simulink model "sim_all"  (R2020a)
settings: Solver=VariableStepAuto  StartTime=0.0  StopTime=2000  RelTol=1e-3
undefined symbols (not defined in the file or in its folder): a1, a2, alpha1, alpha2, cornerA, cornerB, cornerC, cornerD, ctrl_clockwise, ctrl_int_bound_or, ctrl_int_bound_pos, ctrl_k_or, ctrl_k_pos, ctrl_Ki_vel, ctrl_Kp_v_pos, ctrl_Kp_vel, ctrl_TAM, ctrl_Ts, ctrl_va_uncontrolled, ctrl_vel_uncontrolled, D, dead_zone_limit, depth, DiscIntNeverNeededParam, distanceFromWall, initInspectedSide, initPoint, mod_A, mod_Cd_F, mod_Cd_M, mod_eta_init, mod_g, mod_h0, mod_Ixx, mod_Iyy, mod_Izz, mod_Kp_dot, mod_lat0, mod_lon0, mod_m, mod_Mq_dot, mod_ni_init, mod_Nr_dot, mod_p1, mod_p2, mod_p3, mod_p4, mod_p5, mod_p6, mod_R, mod_Rm, mod_t1, mod_t2, mod_t3, mod_t4, mod_t5, mod_t6, mod_W, mod_Xu_dot, mod_Yv_dot ... (+53)
libraries: simulink x8, cstblocks x6, simulink_extras x1
(part 5 of 6)

== matlab function sim_all/Controller_mk4_v3/Mixer/Mix ==
  data: Tp input; T output; Tv input; To input; ctrl_T_max parameter
%% funzione che permette di gestire le saturazioni dei motori
function T = Mix(Tp, Tv, To, ctrl_T_max)
    T_sat = [   ctrl_T_max   ctrl_T_max   ctrl_T_max   ctrl_T_max   ctrl_T_max   ctrl_T_max;...
               -ctrl_T_max  -ctrl_T_max  -ctrl_T_max  -ctrl_T_max  -ctrl_T_max  -ctrl_T_max];
    tmp = Tp + Tv + To;
    freg = sumSat(ctrl_T_max, tmp);                 % freg indica se il vettore è da regolare
    if freg == true
        if sumSat(ctrl_T_max, To+Tp) == false       % caso in cui To+Tp non satura
            T_tmp = To + Tp;
            [T_sat, T_new] = prior(T_sat, T_tmp);
            [T_sat, T_new] = prior(T_sat, Tv);
            T = T_tmp + T_new;
        else                                        % caso generale, ridimensiona tutti i vettori che fanno saturare
            T_tmp = 0;
            [T_sat, T_new] = prior(T_sat, To);
            T_tmp = T_tmp + T_new;
            [T_sat, T_new] = prior(T_sat, Tp);
            T_tmp = T_tmp + T_new;
            [T_sat, T_new] = prior(T_sat, Tv);
            T = T_tmp + T_new;
        end
    else
        T = tmp;
    end
end

% sumSat() restituisce 1 se il vettore T_in supera la saturazione, è solo
% un controllo iniziale in quanto controlla solo se la somma delle spinte
% rientra in T_max
function resp = sumSat(T_max, T_in)
    tmp = false;
    for i=1:length(T_in)
        if abs(T_in(i)) > T_max
            tmp = true;
        end
    end
    resp = tmp;
end

% prior() prende vettore in ingresso e vettore delle saturazioni e
% restituisce vettore in ingresso ridimensionato e nuovo vettore delle
% saturazioni
function [T_sat_new, T_reg] = prior(T_sat, T_new)
    T_sat_tmp = T_sat;
    recalc = false;                 % serve per sapere se bisogna ricalcolare le precedenti saturazioni
    for i = 1:length(T_new)         % ciclo per calcolare i nuovi vettori ridimensionati
        if T_new(i)>0               % azione del motore positiva
            tmp = T_sat_tmp(1,i) - T_new(i);        % nuova saturazione temporanea
            if tmp < 0
                if i < 5                            % devo scalare i primi 4 motori per mantenere la direzione
                    k = abs(T_sat_tmp(1,i)/T_new(i));
                    T_new(1:4) = T_new(1:4) * k;
                    if i~=1                 % devo riaggiustare le T_sat precedenti se il motore che satura non è il primo
                        recalc = true;      % riaggiusto i T_sat in prior2
                    end
                else
                    k = abs(T_sat_tmp(1,i)/T_new(i));
                    j = ((floor(i/2.1)+1)*2);           % escamotage per prendere le coppie giuste, era per le coppie
                    T_new(j-1:j) = T_new(j-1:j) * k;    % ridimensiono le componenti relative al grado di libertà
                    if mod(i, 2) == 0                   % devo riaggiustare la T_sat precedente se i pari
                        recalc = true;                  % riaggiusto gli T_sat
                    end
                end
            end
            T_sat_tmp(1,i) = T_sat_tmp(1,i) - T_new(i);
            T_sat_tmp(2,i) = T_sat_tmp(2,i) - T_new(i);
        elseif T_new(i)<0                           % è identico al codice per T>0 ma speculare
            tmp = T_sat_tmp(2,i) - T_new(i);
            if tmp > 0
                if i < 5                            % devo scalare i primi 4 motori
                    k = abs(T_sat_tmp(2,i)/T_new(i));
                    T_new(1:4) = T_new(1:4) * k;
                    if i~=1                         % devo riaggiustare le T_sat precedenti se i 
                        recalc = true;              % riaggiusto gli T_sat
                    end
                else
                    k = abs(T_sat_tmp(2,i)/T_new(i));
                    j = (floor(i/2.1)+1)*2;     % escamotage per prendere le coppie giuste
                    T_new(j-1:j) = T_new(j-1:j) * k;
                    if mod(i, 2) == 0           % devo riaggiustare la T_sat precedente se i pari
                        recalc = true;          % riaggiusto gli T_sat
                    end
                end
            end
            T_sat_tmp(2,i) = T_sat_tmp(2,i) - T_new(i);
            T_sat_tmp(1,i) = T_sat_tmp(1,i) - T_new(i);
        end
    end
    if recalc == true
        % devo rifare il ciclo con i nuovi T_new
        [T_sat_tmp, T_new] = prior2(T_sat, T_new);
    end
    T_sat_new = T_sat_tmp;      % T_sat_new è il nuovo vettore delle saturazioni
    T_reg = T_new;              % T_reg è il nuovo vettore scalato
end

% prior2() aggiusta il vettore delle saturazioni T_sat, uso interno a
% prior()
function [T_sat_new, T_reg] = prior2(T_sat, T_new)
    T_sat_tmp = T_sat;
    for i = 1:length(T_new)        % ciclo per calcolare quanti giri rimanenti prima di saturare
        if T_new(i)>0              % azione del motore positiva
            tmp = T_sat_tmp(1,i) - T_new(i);       % nuova saturazione temporanea
            T_sat_tmp(1,i) = tmp;
            T_sat_tmp(2,i) = T_sat_tmp(2,i) - T_new(i);
        else
            tmp = T_sat_tmp(2,i) - T_new(i);
            T_sat_tmp(2,i) = tmp;
            T_sat_tmp(1,i) = T_sat_tmp(1,i) - T_new(i);
        end
    end
    T_sat_new = T_sat_tmp;
    T_reg = T_new;
end

== matlab function sim_all/Mission_supervisor_v3/Mission_Supervisor/MATLAB Function1 ==
  data: punto_iniz_patt output size=3; initInspectedSide parameter; distanceFromWall parameter; initPoint parameter; Or_in output; dps_fin output; cornerA parameter; cornerB parameter; cornerC parameter; cornerD parameter; relativeDirection parameter; alfa output
function [punto_iniz_patt, Or_in, dps_fin, alfa] = ambiente(initInspectedSide,distanceFromWall,initPoint,cornerA, cornerB, cornerC, cornerD, relativeDirection)
 
    %% Unità di misura 
    
    % punto_iniz_patt, initPoint, cornerA, cornerB, cornerC, cornerD        [deg, deg, m]
    % Or_in                                                                 [rad, rad, rad]
    % dps_fin,distanceFromWall                                              [m]
    % alfa                                                                  [rad]
    % relativeDirection                                                     [deg]

    %% Inizializzazione variabili
    
    % Valori dati da file relativi agli angoli del bacino
    iP = initPoint;
    A = cornerA;
    B = cornerB;
    C = cornerC;
    D = cornerD;

    coder.extrinsic('evalin', 'wgs84Ellipsoid', 'geodetic2ned');
    coder.extrinsic('evalin', 'wgs84Ellipsoid', 'ned2geodetic');

    % Inizializzazione di alcune variabili
    xA = 0; yA = 0; zA = 0; xB = 0; yB = 0; zB = 0; xC = 0; yC = 0; zC = 0; 
    xD = 0; yD = 0; zD = 0; xiP = 0; yiP = 0; ziP = 0;
    xpipAB = 0; ypipAB = 0; zpipAB = 0; xpipBC = 0; ypipBC = 0; zpipBC = 0; 
    xpipCD = 0; ypipCD = 0; zpipCD = 0; xpipDA = 0; ypipDA = 0; zpipDA = 0;
    depth_in = initPoint(3);
    Or_in = [0; 0; 0];
    
    % Conversione da Geodetic a NED delle posizioni degli angoli e del punto iniziale
    wgs84 = wgs84Ellipsoid; % Per il corretto funzionamento e' necessario installare un 
                            % pacchetto aggiuntivo in Matlab qualora non fosse presente
    [xA, yA, zA] = geodetic2ned(A(1), A(2), 0, C(1), C(2), 0, wgs84);
    [xB, yB, zB] = geodetic2ned(B(1), B(2), 0, C(1), C(2), 0, wgs84);
    [xC, yC, zC] = geodetic2ned(C(1), C(2), 0, C(1), C(2), 0, wgs84);
    [xD, yD, zD] = geodetic2ned(D(1), D(2), 0, C(1), C(2), 0, wgs84);
    [xiP, yiP, ziP] = geodetic2ned(iP(1), iP(2), 0, C(1), C(2), 0, wgs84);
    inizio = [xiP; yiP; depth_in];

    % Punti centrali delle pareti
    pcAB = [(xB + xA)/2; (yB + yA)/2; depth_in];
    pcBC = [(xB + xC)/2; (yB + yC)/2; depth_in];   
    pcCD = [(xC + xD)/2;(yC + yD)/2; depth_in];
    pcDA = [(xD + xA)/2; (yD + yA)/2; depth_in];

    % Lunghezze delle pareti
    AB = sqrt((xA - xB)^2 + (yA - yB)^2); 
    BC = sqrt((xB - xC)^2 + (yB - yC)^2); 
    CD = sqrt((xC - xD)^2 + (yC - yD)^2); 
    DA = sqrt((xD - xA)^2 + (yD - yA)^2); 
    
    dW = distanceFromWall;

    %% Calcolo punto di inizio pattugliamento a meta' parete

    % Calcolo degli angoli relativi tra le pareti 
    thetaBC = acos(yB/BC);          
    thetaCD = acos(yD/CD);
    gammaAB = acos((yB - yA)/AB);
    thetaAB = pi - gammaAB;
    gammaDA = acos((yA - yD)/DA);

    % Punti di inizio pattugliamento a seconda di quale parete è scelta come
    % parete iniziale
    
    dbpc = sqrt((pcAB(1) - xB)^2 + (pcAB(2) - yB)^2);
    hpb = sqrt(dbpc^2 + dW^2);
    alfa1 = - acos(dbpc/hpb);
    gammaab = pi - (gammaAB + alfa1);
    pcab1 = [hpb * sin(gammaab), hpb * cos(gammaab)];
    pipAB = [xB + pcab1(1); yB + pcab1(2); depth_in];

    dcpc = sqrt(pcBC(1)^2 + pcBC(2)^2);
    hpc = sqrt(dcpc^2 + dW^2);
    alfabc = acos(dcpc/hpc);
    gammaBC = thetaBC + alfabc;
    pipBC = [hpc * sin(gammaBC); hpc * cos(gammaBC); depth_in];

    dcdpc = sqrt(pcCD(1)^2 + pcCD(2)^2);
    hpcd = sqrt(dcdpc^2 + dW^2);
    alfacd = acos(dcdpc/hpcd);
    gammaCD = thetaCD - alfacd;
    pipCD = [hpcd * sin(gammaCD); hpcd * cos(gammaCD); depth_in];

    dapc = sqrt((pcDA(1) - xA)^2 + (pcDA(2) - yA)^2);
    hpda = sqrt(dapc^2 + dW^2);
    alfada = acos(dapc/hpda);
    gammada = pi + (gammaDA + alfada);
    pcda1 = [hpda * sin(gammada), hpda * cos(gammada)];
    pipDA = [xA + pcda1(1); yA + pcda1(2); depth_in];
    
    % Si convertono i punti "pip" da NED a Geodetic 
    [xpipAB, ypipAB, zpipAB] = ned2geodetic(pipAB(1), pipAB(2), pipAB(3), C(1), C(2), 0, wgs84);
    [xpipBC, ypipBC, zpipBC] = ned2geodetic(pipBC(1), pipBC(2), pipBC(3), C(1), C(2), 0, wgs84);
    [xpipCD, ypipCD, zpipCD] = ned2geodetic(pipCD(1), pipCD(2), pipCD(3), C(1), C(2), 0, wgs84);
    [xpipDA, ypipDA, zpipDA] = ned2geodetic(pipDA(1), pipDA(2), pipDA(3), C(1), C(2), 0, wgs84);

    pipAB_geodetic = [xpipAB; ypipAB; depth_in];
    pipBC_geodetic = [xpipBC; ypipBC; depth_in];
    pipCD_geodetic = [xpipCD; ypipCD; depth_in];
    pipDA_geodetic = [xpipDA; ypipDA; depth_in];

    %% Calcolo angolo di orientazione iniziale in direzione del punto di inizio  pattugliamento (rispetto al nord)

    % Versore orinetato verso il nord n = [1, 0, 0];
    
    % Vettori che vanno dal punto di partenza al punto di inizio pattugliamento
    
    iAB = pipAB - inizio;
    iBC = pipBC - inizio;
    iCD = pipCD - inizio;
    iDA = pipDA - inizio;

    % Angoli tra direzione Nord e il vettore che porta verso il punto di inizio pattugliamento. 
    % Sono gli angoli di orientazione iniziale desiderata. 
    theta1 = atan2d(iAB(2),iAB(1));
    theta2 = atan2d(iBC(2),iBC(1));
    theta3 = atan2d(iCD(2),iCD(1));
    theta4 = atan2d(iDA(2),iDA(1));
    
    % Si raccoglie in un vettore
    theta = [deg2rad(theta1), deg2rad(theta2), deg2rad(theta3), deg2rad(theta4)];

    %% Si calcolano gli angoli interni dei vertici
    
    alfaC = thetaCD - thetaBC;
    alfaB = pi - (thetaAB-thetaBC);
    alfaA = thetaAB - gammaDA;
    alfaD = 2*pi - alfaA - alfaB - alfaC;
    alfa = [alfaA; alfaB; alfaC; alfaD];    %Utilizzati poi in fase di manovra

    %% Calcolo distanza dalla parete successiva a partire da meta'  parete

    % Sono le distanze da metà parete alla parete successiva
    dABpc = sqrt((pcAB(1) - xB)^2 + (pcAB(2) - yB)^2);
    dBCpc = sqrt(pcBC(1)^2 + pcBC(2)^2);
    dCDpc = sqrt(pcCD(1)^2 + pcCD(2)^2);
    dDApc = sqrt((pcDA(1) - xA)^2 + (pcDA(2) - yA)^2);


    %% Scelta delle condizioni

    % In base al valore di parete iniziale si assegnano i giusti valori per i 
    % riferimenti da utilizzare nei vari stati
    
    if initInspectedSide == 1

        punto_iniz_patt = pipAB_geodetic;
        Or_in = [0; 0; theta(1)];
        dps_fin = dABpc;

    elseif initInspectedSide == 2

        punto_iniz_patt = pipBC_geodetic;
        Or_in = [0; 0; theta(2)];
        dps_fin = dBCpc;

    elseif initInspectedSide == 3

        punto_iniz_patt = pipCD_geodetic;
        Or_in = [0; 0; theta(3)];
        dps_fin = dCDpc;

    else

        punto_iniz_patt = pipDA_geodetic;
        Or_in = [0; 0; theta(4)];
        dps_fin = dDApc;

    end
                                                                            %****TEST*****%
                                                                            %Or_in = [1; 1; 1];

end

== matlab function sim_all/Controller_mk4_v3/Mixer/T2n ==
  data: T input size=[6 1]; n output; a1 parameter
%% Conversione da T a n
% Si usa relazione inclusa nel modello dei propulsiori
% sfruttando approssimazione quadratica
function n = T2n(T,a1)
n = zeros(6,1);
    for i= 1:length(T)
        if T(i) > 0
            n(i) = sqrt(T(i)/a1);
        else
            n(i) = -sqrt(-T(i)/a1);
        end
    end
end

== matlab function sim_all/Controller_mk4_v3/enabler ==
  settings: updateMethod=DISCRETE  sampleTime=ctrl_Ts
  data: state input; en_pos output; en_vel output; en_or output
function [en_pos, en_vel, en_or] = fcn(state)
    en = [0 0 0];
    persistent state_prec        % reset dell'azione integrale
    if isempty(state_prec)
        state_prec = 0;
    end
    if state ~= state_prec
        en = [0 0 0];
        state_prec = state;
    else
        switch state
            case 100            % fermo in superficie
                en = [1 0 0];
            case 101            % orientazione verso parete di inizio in superficie
                en = [1 0 1];
            case 102            % posizionamento in superficie
                en = [1 0 1];   
            case 103            % immersione
                en = [1 0 1];
            case 104            % orientazione in profondità
                en = [1 0 1];
            case 201            % pattugliamento
                en = [1 1 1];
            case 202            % frenata, da verificare con gli altri
                en = [1 0 1];
            case 203            % manovra di cambio parete
                en = [1 0 1];
            case 204            % competamento del pattugliamento della parete iniziale
                en = [1 1 1];
            case 205            % frenata a metà parete
                en = [1 0 1];
            case 301            % risalita
                en = [1 0 1];
            case 302            % orientazione in superficie
                en = [1 0 1];
            case 303            % rientro, ritorno al punto iniziale in superficie
                en = [1 0 1];
            case 304            % fine missione, tutto spento
                en = [0 0 0];
        end
    end
    en_pos = en(1);
    en_vel = en(2);
    en_or = en(3);
end

== matlab function sim_all/Controller_mk4_v3/lld2Ned ==
  data: x_ecef input size=[3 1]; x_n output; cornerC parameter
%% Da LLD (riferimento posizione assoluta) a NED
function x_n = ToNed_Pos(x_ecef,cornerC)
x_n=zeros(3,1);
coder.extrinsic('evalin', 'wgs84Ellipsoid', 'geodetic2ned');
[pNorth,pEast,pDown] = geodetic2ned(x_ecef(1),x_ecef(2),x_ecef(3),cornerC(1),cornerC(2),0,wgs84Ellipsoid);
x_n=[pNorth;pEast;x_ecef(3)];

end

== matlab function sim_all/Model/Vehicle Model/Acceleration Computation ==
  data: inertialTerm input; ni_dot output; mod_m parameter; mod_Ixx parameter; mod_Iyy parameter; mod_Izz parameter; mod_Xu_dot parameter; mod_Yv_dot parameter; mod_Zw_dot parameter; mod_Kp_dot parameter; mod_Mq_dot parameter; mod_Nr_dot parameter
function ni_dot = fcn(inertialTerm, mod_m, mod_Ixx, mod_Iyy, mod_Izz, mod_Xu_dot, mod_Yv_dot, mod_Zw_dot, mod_Kp_dot, mod_Mq_dot, mod_Nr_dot)

% Si definisce la matrice di inerzia del corpo rigido:
Mrb = [ mod_m   0   0   0   0   0;
        0   mod_m   0   0   0   0;
        0   0   mod_m   0   0   0;
        0   0   0  mod_Ixx  0   0;
        0   0   0   0  mod_Iyy  0;
        0   0   0   0   0  mod_Izz ];

% Si definisce la matrice di inerzia dovuta ai termini di massa e inerzia
% aggiunti:
Ma = [ -mod_Xu_dot     0        0        0        0        0;
          0     -mod_Yv_dot     0        0        0        0;
          0        0     -mod_Zw_dot     0        0        0;
          0        0        0     -mod_Kp_dot     0        0;
          0        0        0        0     -mod_Mq_dot     0;
          0        0        0        0        0     -mod_Nr_dot ];

M = Mrb + Ma;

ni_dot = M\inertialTerm;

== matlab function sim_all/Model/Vehicle Model/Coriolis term ==
  data: ni_rel input; mod_m parameter; mod_Ixx parameter; mod_Iyy parameter; mod_Izz parameter; mod_Xu_dot parameter; mod_Yv_dot parameter; mod_Zw_dot parameter; mod_Kp_dot parameter; Cterm output; mod_Mq_dot parameter; mod_Nr_dot parameter
function Cterm  = fcn(ni_rel, mod_m, mod_Ixx, mod_Iyy, mod_Izz, mod_Xu_dot, mod_Yv_dot, mod_Zw_dot, mod_Kp_dot, mod_Mq_dot, mod_Nr_dot)

u_rel = ni_rel(1);
v_rel = ni_rel(2);
w_rel = ni_rel(3);
p_rel = ni_rel(4);
q_rel = ni_rel(5);
r_rel = ni_rel(6);

% Si definisce la matrice di Coriolis del corpo rigido:
Crb = [    0          0          0           0          mod_m*w_rel     -mod_m*v_rel;
           0          0          0       -mod_m*w_rel          0         mod_m*u_rel;
           0          0          0        mod_m*v_rel      -mod_m*u_rel         0;
           0       mod_m*w_rel   -mod_m*v_rel        0        mod_Izz*r_rel   -mod_Iyy*q_rel;
       -mod_m*w_rel       0       mod_m*u_rel   -mod_Izz*r_rel         0       mod_Ixx*p_rel;
        mod_m*v_rel   -mod_m*u_rel       0       mod_Iyy*q_rel   -mod_Ixx*p_rel         0    ];

% Si definiscono i termini di Coriolis dovuti alle masse a alle inerzie
% aggiunte:
Ca = [      0              0              0              0        -mod_Zw_dot*w_rel   mod_Yv_dot*v_rel;
            0              0              0         mod_Zw_dot*w_rel        0        -mod_Xu_dot*u_rel;
            0              0              0        -mod_Yv_dot*v_rel   mod_Xu_dot*u_rel        0;
            0        -mod_Zw_dot*w_rel   mod_Yv_dot*v_rel        0        -mod_Nr_dot*r_rel   mod_Mq_dot*q_rel;
       mod_Zw_dot*w_rel        0        -mod_Xu_dot*u_rel   mod_Nr_dot*r_rel        0        -mod_Kp_dot*p_rel;
      -mod_Yv_dot*v_rel   mod_Xu_dot*u_rel        0        -mod_Mq_dot*q_rel   mod_Kp_dot*p_rel        0       ];

C = Crb + Ca;

Cterm = C*ni_rel;

== matlab function sim_all/Model/Vehicle Model/Damping term ==
  data: ni_rel input; Dterm output; rho parameter; mod_Rm parameter; mod_A parameter; mod_Cd_F parameter; mod_Cd_M parameter
function Dterm = fcn(ni_rel, rho, mod_Rm, mod_A, mod_Cd_F, mod_Cd_M)

u_rel = ni_rel(1);
v_rel = ni_rel(2);
w_rel = ni_rel(3);
p_rel = ni_rel(4);
q_rel = ni_rel(5);
r_rel = ni_rel(6);

%Termine costante di Damping rispettivamente riferito alle forze e ai momenti
Dconst_F = 0.5*rho*mod_Cd_F*mod_A;
Dconst_M = 0.5*rho*mod_Cd_M*mod_A*mod_Rm*mod_Rm*mod_Rm;

% Si definiscono i termini diagonali della matrice di Damping:
D1 = Dconst_F*abs(u_rel)*u_rel;
D2 = Dconst_F*abs(v_rel)*v_rel;
D3 = Dconst_F*abs(w_rel)*w_rel;
D4 = Dconst_M*abs(p_rel)*p_rel;
D5 = Dconst_M*abs(q_rel)*q_rel; 
D6 = Dconst_M*abs(r_rel)*r_rel; 

Dterm = [D1; D2; D3; D4; D5; D6];

== matlab function sim_all/Model/Vehicle Model/Gravitational terms ==
  data: eta input; Gterm output; mod_W parameter; mod_z_cm parameter; mod_R parameter; rho parameter; mod_g parameter
function Gterm = fcn (eta, mod_W, mod_z_cm, mod_R, rho, mod_g)

% Si definisce il vettore delle forze e dei momenti gravitazionali 
% considerando una forza di galleggiamento variabile al variare del volume 
% del veicolo immerso.

z = eta(3);
phi = eta(4);
theta = eta(5);
 
% Si definisce la componente z del vettore posizione del centro di
% galleggiamento rispetto al centro di massa:
z_CB = -0.1;

% Caso di veicolo totalmente immerso:
if (z >= mod_R + mod_z_cm)
    G = [0; 0; 0; mod_z_cm*mod_W*cos(theta)*sin(phi); mod_z_cm*mod_W*sin(theta); 0];

% Caso di veicolo parzialmente immerso (forza di galleggiamento variabile):
elseif (z >= -(mod_R - mod_z_cm) && z < (mod_R + mod_z_cm))
    Vol_immerso = pi*((z+mod_R-mod_z_cm)^2)*(mod_R-((z+mod_R-mod_z_cm)/3));
    B = rho*mod_g*Vol_immerso;
    G = [(mod_W-B)*sin(theta); -(mod_W-B)*cos(theta)*sin(phi); -(mod_W-B)*cos(theta)*cos(phi); -z_CB*B*cos(theta)*sin(phi); -z_CB*B*sin(theta); 0];

% Caso di veicolo completamente emerso (condizione che non si deve verificare per nessun motivo):
else
    G = [mod_W*sin(theta); -mod_W*cos(theta)*sin(phi); -mod_W*cos(theta)*cos(phi); 0; 0; 0];    
end

Gterm = G;

== matlab function sim_all/Model/Vehicle Model/Kinematic Model ==
  data: eta input; ni input; eta_dot output
function eta_dot = fcn(eta, ni)

phi = eta(4);
theta = eta(5); 
psi = eta(6);

% Si definisce la matrice di rotazione J1 che mappa la velocità lineare in 
% terna body nella velocità lineare in terna NED: 
J1 = [ cos(psi)*cos(theta)   -sin(psi)*cos(phi) + (cos(psi)*sin(theta)*sin(phi))   (sin(psi)*sin(phi)) + (cos(psi)*cos(phi)*sin(theta));
       sin(psi)*cos(theta)   (cos(psi)*cos(phi)) + (sin(psi)*sin(theta)*sin(phi))  (-cos(psi)*sin(phi)) + (sin(psi)*sin(theta)*cos(phi));
      -sin(theta)             cos(theta)*sin(phi)                                   cos(theta)*cos(phi)                                  ];

% Si definisce la matrice J2 che mappa la velocità angolare in terna body
% nel vettore orientazione espresso in terna NED (J2 non è una matrice di 
% rotazione):
J2 = [ 1   sin(phi)*tan(theta)   cos(phi)*tan(theta);
       0   cos(phi)             -sin(phi);
       0   sin(phi)/cos(theta)   cos(phi)/cos(theta) ];
       
J = [   J1      zeros(3);
      zeros(3)    J2     ];

eta_dot = J*ni;

== matlab function sim_all/Model/Vehicle Model/P1/Propeller1 ==
  data: n1 input; T1 output; V1 input; D parameter; omega parameter; a1 parameter; a2 parameter; alpha1 parameter; alpha2 parameter
function T1 = thrusterModel(n1, V1, D, omega, a1, a2, alpha1, alpha2)

Va1 = (1-omega) * V1;     % Advancement velocity at the propeller
J0 = Va1/(n1*D);          % Advancement Coefficient

if J0 > -alpha1/alpha2  % Out of linearity domain (right side)
    T1 = 0;              % A null generated thrust is assumed
    
elseif J0 < 0           % Out of linearity domain (left side)
    T1 = a1*abs(n1)*n1;    % Bollard thrust is assumed

else                    % Within the linearity domain
    T1 = a1*abs(n1)*n1 - a2*abs(n1)*V1;
end

== matlab function sim_all/Model/Vehicle Model/P2/Propeller2 ==
  data: n2 input; T2 output; V2 input; D parameter; omega parameter; a1 parameter; a2 parameter; alpha1 parameter; alpha2 parameter
function T2 = thrusterModel(n2, V2, D, omega, a1, a2, alpha1, alpha2)

Va2 = (1-omega) * V2;     % Advancement velocity at the propeller
J0 = Va2/(n2*D);          % Advancement Coefficient

if J0 > -alpha1/alpha2  % Out of linearity domain (right side)
    T2 = 0;              % A null generated thrust is assumed
    
elseif J0 < 0           % Out of linearity domain (left side)
    T2 = a1*abs(n2)*n2;    % Bollard thrust is assumed

else                    % Within the linearity domain
    T2 = a1*abs(n2)*n2 - a2*abs(n2)*V2;
end

== matlab function sim_all/Model/Vehicle Model/P3/Propeller3 ==
  data: n3 input; T3 output; V3 input; D parameter; omega parameter; a1 parameter; a2 parameter; alpha1 parameter; alpha2 parameter
function T3 = thrusterModel(n3, V3, D, omega, a1, a2, alpha1, alpha2)

Va3 = (1-omega) * V3;     % Advancement velocity at the propeller
J0 = Va3/(n3*D);          % Advancement Coefficient

if J0 > -alpha1/alpha2  % Out of linearity domain (right side)
    T3 = 0;              % A null generated thrust is assumed
    
elseif J0 < 0           % Out of linearity domain (left side)
    T3 = a1*abs(n3)*n3;    % Bollard thrust is assumed

else                    % Within the linearity domain
    T3 = a1*abs(n3)*n3 - a2*abs(n3)*V3;
end

== matlab function sim_all/Model/Vehicle Model/P4/Propeller4 ==
  data: n4 input; T4 output; V4 input; D parameter; omega parameter; a1 parameter; a2 parameter; alpha1 parameter; alpha2 parameter
function T4 = thrusterModel(n4, V4, D, omega, a1, a2, alpha1, alpha2)

Va4 = (1-omega) * V4;     % Advancement velocity at the propeller
J0 = Va4/(n4*D);          % Advancement Coefficient

if J0 > -alpha1/alpha2  % Out of linearity domain (right side)
    T4 = 0;              % A null generated thrust is assumed
    
elseif J0 < 0           % Out of linearity domain (left side)
    T4 = a1*abs(n4)*n4;    % Bollard thrust is assumed

else                    % Within the linearity domain
    T4 = a1*abs(n4)*n4 - a2*abs(n4)*V4;
end

== matlab function sim_all/Model/Vehicle Model/P5/Propeller5 ==
  data: n5 input; T5 output; V5 input; D parameter; omega parameter; a1 parameter; a2 parameter; alpha1 parameter; alpha2 parameter
function T5 = thrusterModel(n5, V5, D, omega, a1, a2, alpha1, alpha2)

Va5 = (1-omega) * V5;     % Advancement velocity at the propeller
J0 = Va5/(n5*D);          % Advancement Coefficient

if J0 > -alpha1/alpha2  % Out of linearity domain (right side)
    T5 = 0;              % A null generated thrust is assumed
    
elseif J0 < 0           % Out of linearity domain (left side)
    T5 = a1*abs(n5)*n5;    % Bollard thrust is assumed

else                    % Within the linearity domain
    T5 = a1*abs(n5)*n5 - a2*abs(n5)*V5;
end

== matlab function sim_all/Controller_mk4_v3/C_pos/C_pos_Y ==
  data: err_int output; pos input; vel output; k input; ctrl_vel_uncontrolled parameter; ctrl_int_bound_pos parameter
%% Azione proporzionale
function [err_int, vel] = fcn(pos, k, ctrl_vel_uncontrolled, ctrl_int_bound_pos)
    v = 0;
    err_int = 0;
    vel_des = ctrl_vel_uncontrolled;    % velocità impostata se 'lontani'
    brake_dist = 1/k*vel_des;           % distanza di frenata
    if pos >= brake_dist                % se ho spazio per frenare mantengo la velocità
        v = vel_des;
    end
    if pos <= -brake_dist               % lontani in direzione negativa
        v = -vel_des;
    end
    if  abs(pos) < brake_dist           % se è vicino il proporzionale gestisce la frenata
        v = k*pos;
    end
    vel = v;
    if abs(pos) < ctrl_int_bound_pos    % per il regime può essere utile una azione integrale
        err_int = pos;                  % err_int va ad un integratore
    end

== matlab function sim_all/Model/Vehicle Model/P6/Propeller6 ==
  data: n6 input; T6 output; V6 input; D parameter; omega parameter; a1 parameter; a2 parameter; alpha1 parameter; alpha2 parameter
function T6 = thrusterModel(n6, V6, D, omega, a1, a2, alpha1, alpha2)

Va6 = (1-omega) * V6;     % Advancement velocity at the propeller
J0 = Va6/(n6*D);          % Advancement Coefficient

if J0 > -alpha1/alpha2  % Out of linearity domain (right side)
    T6 = 0;              % A null generated thrust is assumed
    
elseif J0 < 0           % Out of linearity domain (left side)
    T6 = a1*abs(n6)*n6;    % Bollard thrust is assumed

else                    % Within the linearity domain
    T6 = a1*abs(n6)*n6 - a2*abs(n6)*V6;
end

== matlab function sim_all/Model/Vehicle Model/TAM ==
  data: T1 input; tau output; T2 input; T3 input; T4 input; T5 input; T6 input; eta input; mod_R parameter; mod_z_cm parameter
function tau = fcn (T1, T2, T3, T4, T5, T6, eta, mod_R, mod_z_cm)

% Si definisce il vettore delle forze e dei momenti applicati al veicolo al 
% variare dei propulsori immersi o emersi, si assume che i propulsori non 
% funzionino se utilizzati fuori dall'acqua. Si assume inoltre che il
% veicolo esca fuori dall'acqua orizzontalmente (con angoli di pitch e roll
% nulli).

z = eta(3);

% Veicolo completamente immerso, tutti i propulsori funzionano.
if (z >= (mod_R+mod_z_cm)) 
    tau1 = T1 + T2;
    tau2 = T3 + T4;
    tau3 = T5 + T6;
    tau4 = ((-(mod_R+mod_z_cm))*T3) + ((mod_R+mod_z_cm)*T4);
    tau5 = (-mod_R*T5) + (mod_R*T6);
    tau6 = (-mod_R*T1) + (mod_R*T2);
    
% Veicolo emerso in un range che va al dall'estremo superiore fino al 
% centro di massa (il centro di massa è ancora immerso), funzionano tutti i 
% propulsori tranne P4.
elseif (z >= 0 && z < (mod_R+mod_z_cm)) 
    tau1 = T1 + T2;
    tau2 = T3;
    tau3 = T5 + T6;
    tau4 = ((-(mod_R+mod_z_cm))*T3);
    tau5 = (-mod_R*T5) + (mod_R*T6);
    tau6 = (-mod_R*T1) + (mod_R*T2);

% Veicolo immerso in un range che va dall'estremo inferiore fino al centro 
% di massa (il centro di massa è emerso), funziona solo il propulsore P3.
elseif (z >= -(mod_R+mod_z_cm) && z < 0)
    tau1 = 0;
    tau2 = T3;
    tau3 = 0;
    tau4 = ((-(mod_R+mod_z_cm))*T3);
    tau5 = 0;
    tau6 = 0;

% Veicolo completamente emerso, nessun propulsore funziona.
else
    tau1 = 0;
    tau2 = 0;
    tau3 = 0;
    tau4 = 0;
    tau5 = 0;
    tau6 = 0;
end

tau = [tau1; tau2; tau3; tau4; tau5; tau6];

== matlab function sim_all/Model/Vehicle Model/Thruster Velocity Computation ==
  data: V1 output; V2 output; V3 output; V4 output; V5 output; V6 output; ni_rel input; mod_p1 parameter; mod_p2 parameter; mod_p3 parameter; mod_p4 parameter; mod_p5 parameter; mod_p6 parameter; mod_t1 parameter; mod_t2 parameter; mod_t3 parameter; mod_t4 parameter; mod_t5 parameter; mod_t6 parameter
function [V1, V2, V3, V4, V5, V6] = fcn(ni_rel, mod_p1, mod_p2, mod_p3, mod_p4, mod_p5, mod_p6, mod_t1, mod_t2, mod_t3, mod_t4, mod_t5, mod_t6)

% Si spezza il vettore velocità relativa nella componente lineare e angolare:
ni1_rel = [ni_rel(1); ni_rel(2); ni_rel(3)];
ni2_rel = [ni_rel(4); ni_rel(5); ni_rel(6)];

% Si definiscono i vettori velocità dei propulsori: 
Vp1 = ni1_rel + cross(ni2_rel, mod_p1);
Vp2 = ni1_rel + cross(ni2_rel, mod_p2);
Vp3 = ni1_rel + cross(ni2_rel, mod_p3);
Vp4 = ni1_rel + cross(ni2_rel, mod_p4);
Vp5 = ni1_rel + cross(ni2_rel, mod_p5);
Vp6 = ni1_rel + cross(ni2_rel, mod_p6);

% Si proiettano tali velocità lungo le direzioni date dai versori:
V1 = dot(Vp1, mod_t1); 
V2 = dot(Vp2, mod_t2);
V3 = dot(Vp3, mod_t3);
V4 = dot(Vp4, mod_t4);
V5 = dot(Vp5, mod_t5);
V6 = dot(Vp6, mod_t6);

== matlab function sim_all/Model/Vehicle Model/seaCurrent from NED to body ==
  data: seaCurrent_Velocity output; eta input; seaCurrent parameter
function seaCurrent_Velocity = fcn(eta, seaCurrent)

phi = eta(4);
theta = eta(5); 
psi = eta(6);

% Si definisce la matrice di rotazione J1 che mappa la velocità lineare 
% della corrente in terna body nella velocità lineare della corrente in 
% terna NED: 
J1 = [ cos(psi)*cos(theta)   -sin(psi)*cos(phi) + (cos(psi)*sin(theta)*sin(phi))   (sin(psi)*sin(phi)) + (cos(psi)*cos(phi)*sin(theta));
       sin(psi)*cos(theta)   (cos(psi)*cos(phi)) + (sin(psi)*sin(theta)*sin(phi))  (-cos(psi)*sin(phi)) + (sin(psi)*sin(theta)*cos(phi));
      -sin(theta)             cos(theta)*sin(phi)                                   cos(theta)*cos(phi)                                  ];

% Si definisce la matrice J1 inversa in maniera tale da mappare la velocità
% della corrente in terna NED nella velocità lineare della corrente in
% terna body (essendo J1 una matrice di rotazione l'inversa coincide con la
% trasposta):
J1_inv = J1';

%si definisce la velocità della corrente espressa in terna Body
seaCurrent_body = J1_inv*seaCurrent;
seaCurrent_Velocity = [seaCurrent_body; 0; 0; 0];

== matlab function sim_all/Model/from NED to ECEF ==
  data: eta1 input; eta1_ECEF output; mod_lat0 parameter; mod_lon0 parameter; mod_h0 parameter
function eta1_ECEF = fcn(eta1, mod_lat0, mod_lon0, mod_h0)

eta1_ECEF = [0; 0; 0];

eta1_North = eta1(1);
eta1_East = eta1(2);
eta1_Down = eta1(3);

coder.extrinsic('evalin','wgs84Ellipsoid','ned2geodetic')

[lat_ECEF, lon_ECEF, h_ECEF] = ned2geodetic(eta1_North, eta1_East, eta1_Down, mod_lat0, mod_lon0, mod_h0, wgs84Ellipsoid);

eta1_ECEF = [lat_ECEF; lon_ECEF; h_ECEF];

== matlab function sim_all/Sensors/BLOCCO GYRO1/Subsystem/GEOD to NED ==
  data: Bias_G output; t input
function Bias_G  = fcn(t)
ramp=t*(3.8785e-05);
Bias_G=ramp;

== matlab function sim_all/Controller_mk4_v3/C_pos/abs_integrator2/Body2Ned ==
  data: x_b input size=[3 1]; x_n output size=[3 1]; or input
%% Da BODY a NED per integrazione assoluta
function x_n = body2ned(x_b,or)
C=zeros(3,3);
C=Cx(or(1))'*Cy(or(2))'*Cz(or(3))';
x_n = C*x_b;
end

== matlab function sim_all/Controller_mk4_v3/C_pos/abs_integrator2/Ned2Body1 ==
  data: x_n input size=[3 1]; x_b output size=[3 1]; or input
%% Da NED a BODY
function x_b = ned2body(x_n,or)
C=zeros(3,3);
C=Cx(or(1))'*Cy(or(2))'*Cz(or(3))';
x_b = C'*x_n;
end

== matlab function sim_all/Controller_mk4_v3/C_pos/abs_integrator1/Body2Ned ==
  data: x_b input size=[3 1]; x_n output size=[3 1]; or input
%% Da BODY a NED
function x_n = body2ned(x_b,or)
C=zeros(3,3);
C=Cx(or(1))'*Cy(or(2))'*Cz(or(3))';
x_n = C*x_b;
end

== matlab function sim_all/Controller_mk4_v3/C_pos/abs_integrator1/Ned2Body1 ==
  data: x_n input size=[3 1]; x_b output size=[3 1]; or input
%% Da NED a BODY
function x_b = ned2body(x_n,or)
C=zeros(3,3);
C=Cx(or(1))'*Cy(or(2))'*Cz(or(3))';
x_b = C'*x_n;
end

== matlab function sim_all/Mission_supervisor_v3/Mission_Supervisor/Inizio/MATLAB Function ==
  data: current_state output; parete_attuale output; stato_interno output; Pos_d output size=3; Pos_s input; error_flag input; attesa input; initInspectedSide parameter; initPoint parameter; timer parameter; SOS parameter
function [current_state, parete_attuale, stato_interno, Pos_d] =  Inizio(Pos_s, error_flag, attesa, initInspectedSide, initPoint, timer, SOS)
    
    disp("Inizio");
    
    %% Unita' di misura
    
    % Pos_d, Pos_s, initPoint                                                [deg, deg, m]
    % attesa, timer                                                          [s]
    
    %% Inizializzazione variabili
    
    % Mantenimento di stato_interno al valore
    % desiderato durante la permanenza del sistema nello stato corrente.
    stato_interno = 100;

    % Se non si ricevono dati dal GPS per un tempo superiore ad una soglia
    % massima di attesa, la missione viene interrotta poiché non è
    % possibile localizzarsi nel bacino
    if ((isnan(Pos_s(1)) || isnan(Pos_s(2))) && (attesa > timer))
        SOS = 1;
        disp("EMERGENZA: mancata ricezione dati da GPS");
    end
    
    %% Preparazione dei riferimenti 
    
        % Parete di inizio pattugliamento
        parete_attuale = initInspectedSide;
        
        % Posizione di inizio missione
        Pos_d = initPoint; 
        
        
    %% Transizione di stato effettiva
    
        % Quando i riferimenti sono correttamente settati
        % viene comunicato agli altri moduli il passaggio di stato
        current_state = 100;  
        
    %% Decisione dello stato successivo
    
     if error_flag == 1
        disp("EMERGENZA: errore segnalato dagli altri sottosistemi");
        SOS = 1;
     end
    
    % Si verifica lo stato di emergenza e la ricezione di misure dal GPS
    if (SOS == 0 && ((isnan(Pos_s(1)) == false && isnan(Pos_s(2)) == false))) 
        
        stato_interno = 101;   % Si passa allo stato successivo
    else
        if SOS == 1
           
            stato_interno = 304; % Politica di emergenza: si passa in fine missione   
        end
    end

end

== matlab function sim_all/Controller_mk4_v3/C_vel/abs_integrator/Body2Ned ==
  data: x_b input size=[3 1]; x_n output size=[3 1]; or input
%% Da BODY a NED
function x_n = body2ned(x_b,or)
C=zeros(3,3);
C=Cx(or(1))'*Cy(or(2))'*Cz(or(3))';
x_n = C*x_b;
end

== matlab function sim_all/Controller_mk4_v3/C_vel/abs_integrator/Ned2Body1 ==
  data: x_n input size=[3 1]; x_b output size=[3 1]; or input
%% Da NED a BODY
function x_b = ned2body(x_n,or)
C=zeros(3,3);
C=Cx(or(1))'*Cy(or(2))'*Cz(or(3))';
x_b = C'*x_n;
end

== matlab function sim_all/Mission_supervisor_v3/Mission_Supervisor/Risalita/MATLAB Function ==
  data: delta_SOS input; delta_current_ris output; delta_stato_ris output; Pos_d output size=3; Dpp_d output; Dps_d output; Pos_s input; Dpp_s input; Orp_s input; Dps_s input; distanceFromWall parameter; Orp_d output; relativeDirection parameter; soglia_pos parameter; SOS parameter; Dps_fin input; soglia_SOS_pos_ris parameter; soglia_SOS_orp parameter; error_flag input; SOS_205 input; initPoint parameter; soglia_SOS_collisione parameter
function [delta_current_ris, delta_stato_ris, Pos_d, Dpp_d, Dps_d, Orp_d ] = Risalita(delta_SOS, Pos_s, Dpp_s, Orp_s, Dps_s, distanceFromWall, relativeDirection, soglia_pos, SOS, Dps_fin, soglia_SOS_pos_ris, soglia_SOS_orp, error_flag, SOS_205, initPoint, soglia_SOS_collisione)

    disp("Risalita");
    
    %% Unità di misura 
    
    % Pos_d, Pos_s, soglia_pos, initPoint                                                                      [deg,deg,m]
    % Orp_d, Orp_s, soglia_SOS_orp                                                                             [rad]
    % relativeDirection                                                                                        [deg]
    % Dpp_d, Dps_d, Dpp_s, Dps_s, Dps_fin, distanceFromWall, soglia_SOS_collisione_s, soglia_SOS_collisione    [m]

    %% Inizializzazione variabili
    
    delta_stato_ris = 0;
    
    pronti = false; 
    
    %% Preparazione dei riferimenti da fornire ai blocchi successivi
    
    % Posizione da raggiungere
    Pos_d = [nan; nan; initPoint(3)];
    
    % Distanza da mantenere
    Dpp_d = distanceFromWall;
    Dps_d = Dps_fin;
    
    % Orientazione da mantenere
    Orp_d = deg2rad(relativeDirection);
    
    % Transizione di stato effettiva
    delta_current_ris = 301 - delta_SOS;  
    
    
    %% Verifica
    
    % Verifica sull'orientazione rispetto alla parete
    if (abs(Orp_s - Orp_d) > soglia_SOS_orp)
        
        SOS = 1;
        disp("EMERGENZA: Rilevato errore nell'orientazione relativa da parete");
        
    end
                                                                            %******TEST******
                                                                            %test = 30;
    % In base al meccanismo del "gestore dell'emergenza" si distinguono due casi: 
    % uno in cui lo stato di Risalita viene attivato al termine di un 
    % pattugliamento corretto (la codifica dello stato precedente è pari a 205) 
    % ed uno se la transizione in questo stato è dovuta all'aver
    % intrapreso una manovra di emergenza (lo stato precedente è
    % inferiore a 205).
    
    % Si proviene da un pattugliamento senza emergenza e si verifica di 
    % effettuare la risalita nella posizione giusta
    if (delta_SOS == 205 && SOS_205 == 0)
        if (abs(Dpp_s - Dpp_d) > soglia_SOS_pos_ris || ...                                          
            abs(Dps_s - Dps_fin) > soglia_SOS_pos_ris)
             
            SOS = 1;
            disp("EMERGENZA: Avvicinamento eccessivo alla parete");
            
        end
    
    % Si proviene da una situazione di emergenza oppure l'emergenza avviene in
    % "risalita". Verifica di effettuare la risalita senza collisione
    % con le pareti
    elseif (delta_SOS < 205 || SOS_205 == 1)
        
        if (abs(Dpp_s - Dpp_d) > soglia_SOS_collisione || ...
            abs(Dps_s) < soglia_SOS_collisione)
       
            SOS = 1;
            disp("EMERGENZA: Avvicinamento eccessivo alla parete");
            
        end
        
    end
    
    if error_flag == 1
        disp("EMERGENZA: Errore segnalato dagli altri sottosistemi");
        SOS = 1;
    end
    
                                                                            %*****TEST******% 
                                                                            %Dps_fin = 8;

    % Si verifica di aver raggiunto la superficie
    if (SOS == 0 && ... 
        abs(Pos_s(3) - Pos_d(3)) < soglia_pos(3)) 
    
          pronti = true;
        
    end
    
    
    %% Decisione dello stato successivo
    
    if ((pronti == true && (delta_SOS < 205 || SOS_205 == 1) || ...
        (SOS == 1)))
           
           delta_stato_ris = 304 - 301; % Transizione nello stato finale a causa di emergenza
    else
        if pronti == true
            
            delta_stato_ris = 302 - 301; % Transizione eseguita correttamente
        end
    end
    % Si rimane nello stato corrente
     
end

== matlab function sim_all/Controller_mk4_v3/lld2Ned1 ==
  data: x_ecef input size=[3 1]; x_n output; cornerC parameter
%% Da LLD (stima posizione assoluta) a NED
function x_n = ToNed_Pos(x_ecef,cornerC)
x_n=zeros(3,1);
coder.extrinsic('evalin', 'wgs84Ellipsoid', 'geodetic2ned');
[pNorth,pEast,pDown] = geodetic2ned(x_ecef(1),x_ecef(2),x_ecef(3),cornerC(1),cornerC(2),0,wgs84Ellipsoid);
x_n=[pNorth;pEast;x_ecef(3)];

end

== matlab function sim_all/Sensors/Environment and Sensors Model3/MATLAB Function1 ==
  data: pos input; plane_AB input; plane_BC input; plane_CD input; plane_DA input; plane_W input; dist output; Roll input; Pitch input; Yaw input
function dist = inter(pos,plane_AB,plane_BC,plane_CD,plane_DA,plane_W,Roll,Pitch, Yaw)
Nc=3; %numero di campioni per 'croce' di raggio del cono
WBr=deg2rad(5); % ampiezza semifascio del sonar (fascio considerato di 10°)
dist2=zeros(3,3);
R=linspace(Roll-WBr,Roll+WBr,Nc);
P=Pitch;
Y=linspace(Yaw-WBr, Yaw+WBr,Nc);
for j=1:Nc  %costruisco la croce (doppia)
for i=1:Nc
    
R_x = [1        0              0; %roll
      0 cos(R(i))  sin(R(i));
      0 -sin(R(i)) cos(R(i))];
  
R_y = [cos(P) 0 -sin(P); %pitch
          0           1         0;
       sin(P) 0 cos(P)];
   
R_z = [cos(Y(j)) sin(Y(j)) 0; %yaw
      -sin(Y(j)) cos(Y(j)) 0;
          0                 0        1];
      
jaco = (R_z'*R_y');
jacob = jaco*R_x';

    versore_son_body = [0 1 0]';
    versore_son_NED = jacob*versore_son_body;         %versore terna NED sonar prua

    %imposto il sistema per trovare l'intersezione tra la retta con direzione
    %nota e uno dei piani delle pareti del bacino

    t_AB = -(pos(1)+plane_AB(2)*pos(2)+plane_AB(4))/(plane_AB(2)*versore_son_NED(2)+versore_son_NED(1));
    t_BC = -(pos(1)+plane_BC(2)*pos(2)+plane_BC(4))/(plane_BC(2)*versore_son_NED(2)+versore_son_NED(1));
    t_CD = -(pos(1)+plane_CD(2)*pos(2)+plane_CD(4))/(plane_CD(2)*versore_son_NED(2)+versore_son_NED(1));
    t_DA = -(pos(1)+plane_DA(2)*pos(2)+plane_DA(4))/(plane_DA(2)*versore_son_NED(2)+versore_son_NED(1));
    t_W = -(plane_W(3)*pos(3)/(plane_W(3)*versore_son_NED(3)+versore_son_NED(3)));
    
    
    if t_AB < 0
        t_AB = inf;
    end
    if t_BC < 0
        t_BC = inf;
    end
    if t_CD < 0
        t_CD = inf;
    end
    if t_DA < 0
        t_DA = inf;
    end
    if t_W < 0
        t_W = inf;
    end
           dist1 = min([t_AB t_BC t_CD t_DA t_W]);
           
           if dist1==t_W %se incontro l'acqua metto NaN nella misura delle distanze
               dist2(i,j)=NaN;
           else
               dist2(i,j)=dist1;
           end
           
end
end
    contr=isnan(dist2); %controlla la presenza di NaN nel vettore di misure
    sum1=sum(sum(contr)); % conta il numero di NaN presenti
    
    if sum1>4 %incontro un numero di Nan superiore a 4
        dist=NaN;
    else
        dist=mean(nanmean(dist2));
    end
end

== matlab function sim_all/Sensors/Environment and Sensors Model4/MATLAB Function1 ==
  data: pos input size=[3]; plane_AB input; plane_BC input; plane_CD input; plane_DA input; plane_W input; dist output; Roll input; Pitch input; Yaw input
function dist = inter(pos,plane_AB,plane_BC,plane_CD,plane_DA,plane_W,Roll,Pitch, Yaw)
Nc=3; %numero di campioni per 'croce' di raggio del cono=1
WBr=deg2rad(5); % ampiezza semifascio del sonar (fascio considerato di 10°)
dist2=zeros(3,3);
R=linspace(Roll-WBr,Roll+WBr,Nc);
P=Pitch;
Y=linspace(Yaw-WBr, Yaw+WBr,Nc);
for j=1:Nc  %costruisco la croce (doppia)
for i=1:Nc
    
R_x = [1        0              0; %roll
      0 cos(R(i))  sin(R(i));
      0 -sin(R(i)) cos(R(i))];
  
R_y = [cos(P) 0 -sin(P); %pitch
          0           1         0;
       sin(P) 0 cos(P)];
   
R_z = [cos(Y(j)) sin(Y(j)) 0; %yaw
      -sin(Y(j)) cos(Y(j)) 0;
          0                 0        1];
      
jaco = (R_z'*R_y');
jacob = jaco*R_x';

    versore_son_body = [0 -1 0]';
    versore_son_NED = jacob*versore_son_body;         %versore terna NED sonar prua

    %imposto il sistema per trovare l'intersezione tra la retta con direzione
    %nota e uno dei piani delle pareti del bacino

    t_AB = -(pos(1)+plane_AB(2)*pos(2)+plane_AB(4))/(plane_AB(2)*versore_son_NED(2)+versore_son_NED(1));
    t_BC = -(pos(1)+plane_BC(2)*pos(2)+plane_BC(4))/(plane_BC(2)*versore_son_NED(2)+versore_son_NED(1));
    t_CD = -(pos(1)+plane_CD(2)*pos(2)+plane_CD(4))/(plane_CD(2)*versore_son_NED(2)+versore_son_NED(1));
    t_DA = -(pos(1)+plane_DA(2)*pos(2)+plane_DA(4))/(plane_DA(2)*versore_son_NED(2)+versore_son_NED(1));
    t_W = -(plane_W(3)*pos(3)/(plane_W(3)*versore_son_NED(3)+versore_son_NED(3)));
    
    
    if t_AB < 0
        t_AB = inf;
    end
    if t_BC < 0
        t_BC = inf;
    end
    if t_CD < 0
        t_CD = inf;
    end
    if t_DA < 0
        t_DA = inf;
    end
    if t_W < 0
        t_W = inf;
    end
           dist1 = min([t_AB t_BC t_CD t_DA t_W]);
           
           if dist1==t_W %se incontro l'acqua metto NaN nella misura delle distanze
               dist2(i,j)=NaN;
           else
               dist2(i,j)=dist1;
           end
           
end
end
    contr=isnan(dist2); %controlla la presenza di NaN nel vettore di misure
    sum1=sum(sum(contr)); % conta il numero di NaN presenti
    
    if sum1>4 %incontro un numero di Nan superiore a 4
        dist=NaN;
    else
        dist=mean(nanmean(dist2));
    end
end

== matlab function sim_all/Sensors/Environment and Sensors Model6/MATLAB Function1 ==
  data: pos input; plane_AB input; plane_BC input; plane_CD input; plane_DA input; plane_W input; dist output; Roll input; Pitch input; Yaw input
function dist = inter(pos,plane_AB,plane_BC,plane_CD,plane_DA,plane_W,Roll,Pitch, Yaw)
Nc=3; %numero di campioni per 'croce' di raggio del cono
WBr=deg2rad(5); % ampiezza semifascio del sonar (fascio considerato di 10°)
dist2=zeros(3,3);
R=Roll;
P=linspace(Pitch-WBr,Pitch+WBr,Nc);
Y=linspace(Yaw-WBr, Yaw+WBr,Nc);

for j=1:Nc  %costruisco la croce (doppia)
for i=1:Nc
    
R_x = [1        0              0; %roll
      0 cos(R)  sin(R);
      0 -sin(R) cos(R)];
  
R_y = [cos(P(i)) 0 -sin(P(i)); %pitch
          0           1         0;
       sin(P(i)) 0 cos(P(i))];
   
R_z = [cos(Y(j)) sin(Y(j)) 0; %yaw
      -sin(Y(j)) cos((j)) 0;
          0                 0        1];
      
jaco = (R_z'*R_y');
jacob = jaco*R_x';

    versore_son_body = [1 0 0]'; %prua
    versore_son_NED = jacob*versore_son_body;         %versore terna NED sonar prua

    %imposto il sistema per trovare l'intersezione tra la retta con direzione
    %nota e uno dei piani delle pareti del bacino

    t_AB = -(pos(1)+plane_AB(2)*pos(2)+plane_AB(4))/(plane_AB(2)*versore_son_NED(2)+versore_son_NED(1));
    t_BC = -(pos(1)+plane_BC(2)*pos(2)+plane_BC(4))/(plane_BC(2)*versore_son_NED(2)+versore_son_NED(1));
    t_CD = -(pos(1)+plane_CD(2)*pos(2)+plane_CD(4))/(plane_CD(2)*versore_son_NED(2)+versore_son_NED(1));
    t_DA = -(pos(1)+plane_DA(2)*pos(2)+plane_DA(4))/(plane_DA(2)*versore_son_NED(2)+versore_son_NED(1));
    t_W = -(plane_W(3)*pos(3)/(plane_W(3)*versore_son_NED(3)+versore_son_NED(3)));
    
    
    if t_AB < 0
        t_AB = inf;
    end
    if t_BC < 0
        t_BC = inf;
    end
    if t_CD < 0
        t_CD = inf;
    end
    if t_DA < 0
        t_DA = inf;
    end
    if t_W < 0
        t_W = inf;
    end
           dist1 = min([t_AB t_BC t_CD t_DA t_W]);
           
           if dist1==t_W %se incontro l'acqua metto NaN nella misura delle distanze
               dist2(i,j)=NaN;
           else
               dist2(i,j)=dist1;
           end
           
end
end
    contr=isnan(dist2); %controlla la presenza di NaN nel vettore di misure
    sum1=sum(sum(contr)); % conta il numero di NaN presenti
    
    if sum1>4 %incontro un numero di Nan superiore a 4
        dist=NaN;
    else
        dist=mean(nanmean(dist2));
    end
end
